simulink library "solar_panels_lib"  (R2018b)
settings: Solver=VariableStepAuto  StartTime=0.0  StopTime=10.0  RelTol=1e-3
libraries: aerolibutil x1
settings Model: Creator=Taylor  LastModifiedBy=Taylor

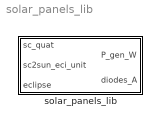
== system solar_panels_lib ==
  solar_panels_lib : Subsystem

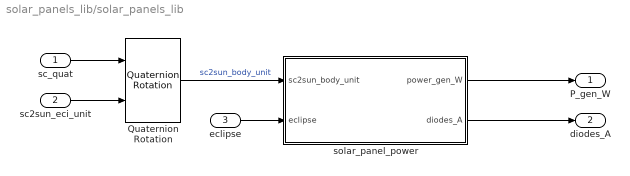
== system solar_panels_lib/solar_panels_lib ==
  sc_quat : Inport
  sc2sun_eci_unit : Inport  Port=2
  eclipse : Inport  Port=3
  Quaternion Rotation : aerolibutil/Quaternion Rotation
  solar_panel_power : MATLAB Function  TreatAsAtomicUnit=on
  P_gen_W : Outport
  diodes_A : Outport  Port=2
  wires:
  sc_quat/1 -> Quaternion Rotation/1
  sc2sun_eci_unit/1 -> Quaternion Rotation/2
  Quaternion Rotation/1 -> solar_panel_power/1(sc2sun_body_unit)  "sc2sun_body_unit"
  solar_panel_power/1(power_gen_W) -> P_gen_W/1
  solar_panel_power/2(diodes_A) -> diodes_A/1
  eclipse/1 -> solar_panel_power/2(eclipse)

== matlab function solar_panels_lib/solar_panel_power ==
  data: sc2sun_body_unit input; eclipse input; power_gen_W output; simParams parameter; diodes_A output
function [power_gen_W,diodes_A] = get_power_gen(sc2sun_body_unit,eclipse,simParams)
%GET_POWER_GEN
% 
% get_power_gen(sc2sun_body_unit,simParams) computes the total power being
% generated by the solar panels located on each of face. Assumes power
% generation is proportional to the square of the cosine of the incidence 
% angle to the sun, and can generate a maximum of 'maxPower' for each face.
%
% Assumes there are solar panels on all 6 sides of cuboid s/c, but fewer
% faces can be modeled by setting the 'maxPower' of those faces to zero.
% ORDER OF FACES: [ +x, -x, +y, -y, +z, -z ]
%
% This function also outputs the current reading from the photodiode on
% each face in Amps as diodes_A
%
% T. Reynolds
%#codegen

power_gen_W = zeros(6,1);
diodes_A    = zeros(6,1);

if (eclipse)
    return;
else
    normals     = simParams.sensors.solar_panels.normals;
    maxPower    = simParams.sensors.solar_panels.maxPower;
    I_out_ApW   = simParams.sensors.photodiodes.I_out_ApW;
    
    for k = 1:6
        % compute cos(incidence)
        sdotf = dot(normals(:,k),sc2sun_body_unit);
        cinc  = saturate(sdotf);
        
        % compute power generated on ith face
        power_gen_W(k) = maxPower(k) * cinc * cinc;
        
        % compute photodiode current
        diodes_A(k) = power_gen_W(k) * I_out_ApW;
    end
    
end

end

function y = saturate(x)
    if( x < 0 )
        y = 0.0;
    elseif( x >= 1.0 )
        y = 1.0;
    else
        y = x;
    end
end
